simulink model "Super11V2_tmp"  (Simulink 8.3)
settings: Solver=FixedStepDiscrete  StartTime=0.0  StopTime=10.0  RelTol=1e-3
settings Model: Creator=scaife  LastModifiedBy=bourbouh  CovSFcnEnable=on  ExtModeAutoUpdateStatusClock=off
settings DataIOCC: SignalLoggingName=sigsOut
settings DebuggingCC: SaveWithParameterizedLinksMsg=none  SignalResolutionControl=TryResolveAllWithWarning  SolverPrmCheckMsg=none  MultiTaskDSMMsg=warning  MultiTaskCondExecSysMsg=none  FrameProcessingCompatibilityMsg=error  StateNameClashWarn=none
settings HardwareCC: TargetBitPerLong=64  TargetBitPerPointer=64  TargetLongLongMode=on  TargetIntDivRoundTo=Zero  TargetEndianess=LittleEndian  TargetWordSize=64  TargetHWDeviceType=MATLAB Host  ProdEqTarget=off
settings SFSimCC: SimParseCustomCode=off
settings RTWCC: SystemTargetFile=rsim.tlc  TemplateMakefile=rsim_default_tmf  Description=Rapid Simulation Target
settings RSimTargetCC: ERTMultiwordTypeDef=System defined  ERTMultiwordLength=256  GeneratePreprocessorConditionals=Use local settings

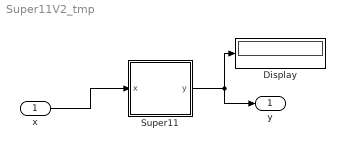
== system Super11V2_tmp ==
  x : Inport
  Display : Display
  Super11 : Stateflow chart  TreatAsAtomicUnit=on
      settings: PermitHierarchicalResolution=ParametersOnly
  y : Outport
  wires:
  x/1 -> Super11/1(x)
  Super11/1(y) -> Display/1, y/1

== stateflow chart Super11 ==
  state A
    du : y++;
  state B
    du : y++;
    state B1
      du : y++;
    state B2
      du : y++;
      state B2a
        du : y++;
      (default) -> B2a
      B2a -> (junction 11)
    (default) -> B1
    B1 -> B2
    (junction 11) -> B1 [order 2] : [x<>0]
  (junction 16) -> B [order 1] : [x==0]
  A -> (junction 16)
  (junction 16) -> B2a [order 2] : [x<>0]
  (junction 11) -> A [order 1] : [x==0]
  (default) -> A
  data: x input int8; y output int32
